simulink model "ErikSchneider_prj_2_5_task1"  (R2025a)
settings: Solver=VariableStepAuto  StartTime=0.0  StopTime=10.0  RelTol=1e-3
settings Model: Creator=eriks  LastModifiedBy=eriks

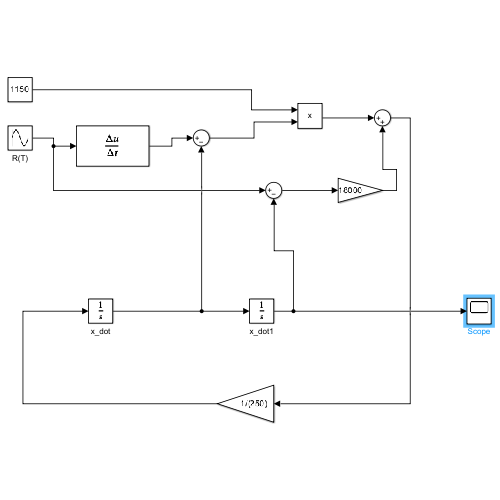
[thumbnail: Simulink's stored preview of the top-level diagram]
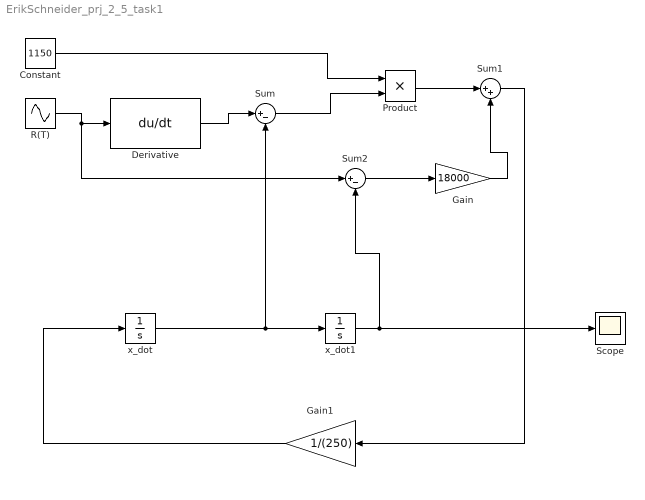
== system ErikSchneider_prj_2_5_task1 ==
  Constant : Constant  Value=1150
  Derivative : Derivative
  Gain : Gain  Gain=18000
  Gain1 : Gain  Gain=1/(250)
  Product : Product
  R(T) : Sin  Amplitude=0.01  Frequency=10  SampleTime=0
  Scope : Scope
      settings: ActiveDisplayYMinimum=-0.029001046028063752  ActiveDisplayYMaximum=0.038299683111001542
  Sum : Sum  Inputs=|+-
  Sum1 : Sum  Inputs=|++
  Sum2 : Sum  Inputs=|+-
  x_dot : Integrator
  x_dot1 : Integrator
  wires:
  Constant/1 -> Product/1
  R(T)/1 -> Sum2/1, Derivative/1
  Derivative/1 -> Sum/1
  Sum/1 -> Product/2
  x_dot/1 -> Sum/2, x_dot1/1
  Gain1/1 -> x_dot/1
  Sum2/1 -> Gain/1
  x_dot1/1 -> Scope/1, Sum2/2
  Sum1/1 -> Gain1/1
  Gain/1 -> Sum1/2
  Product/1 -> Sum1/1
